simulink model "amp_qpsk"  (Simulink 6.0)
settings: Solver=FixedStepDiscrete  StartTime=0.0  StopTime=10.0  RelTol=1e-3
undefined symbols (not defined in the file or in its folder): read, rfdata
libraries: rfports1 x2, commfilt2 x2, commsink2 x2, rfamplifiers1 x1, commdigbbndpm2 x1, commrandsrc2 x1, simulink x1
settings Model: Creator=ashivapr  LastModifiedBy=fwei  ProdHWDeviceType=Specified
settings DataIOCC: SaveOutput=off  SaveTime=off  SignalLoggingName=logsOut
settings DebuggingCC: CheckExecutionContextPreStartOutputMsg=on  CheckExecutionContextRuntimeOutputMsg=on  SolverPrmCheckMsg=none  InheritedTsInSrcMsg=none
settings HardwareCC: ProdHWDeviceType=Specified
settings ModelReferenceCC: UpdateModelReferenceTargets=IfOutOfDate

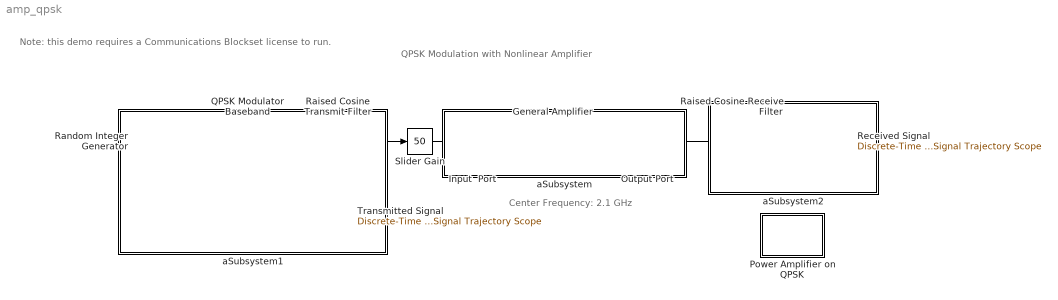
== system amp_qpsk ==
  note: QPSK Modulation with Nonlinear Amplifier
  note: Center Frequency: 2.1 GHz
  note: Note: this demo requires a
      | Communications Blockset
      | license to run.
  General Amplifier : rfamplifiers1/General Amplifier  PhysicalDomain=rfsystemsdomain  SubClassName=general-amplifier  LeftPortType=p1  RightPortType=p1  LConnTagsString=__newl0  RConnTagsString=__newr0  RFDATA=read(rfdata.data, 'default.amp')  InterpMethod=Cubic  IP3Type=OIP3  IIP3=inf  OIP3=inf  NF=0  DisplayData=off  PlotFreq=Derived from Input Port parameters  PlotFreqNoSim=Extracted from RFDATA object  Freq=[1.0e9:1.0e8:2.9e9]  AllPlotType=X-Y plane  NetworkData=S21  PowerData=S11  SmithData=S11  PolarData=S11  ComplexFormat=Magnitude (decibels)  DBFormat=Magnitude (decibels)  PowerFormat=dBm  PhaseFormat=Angle (degrees)  NoneFormat=None
  Input  Port : rfports1/Input Port  Description=source block  MaxLength=128  Fc=2.1e9  Ts=3e-9/8  Zs=50  NoiseFlag=off  seed=67987  GoToTag=AABDAKNBHBUINLASQGFHOGA
  Output Port : rfports1/Output Port  Zl=50  num_Models=3  GoToTag=AABDAKNBHBUINLASQGFHOGA  DisplayData=off  PlotFreq=Derived from Input Port parameters  Freq=1e9:1e8:3e9  AllPlotType=Composite data  NoBudgetPlot=Composite data  NetworkData=S11  SmithData=S11  PolarData=S11  ComplexFormat=Magnitude (decibels)  DBFormat=Magnitude (decibels)  DBMFormat=dBm  NoneFormat=None
  Power Amplifier on QPSK : Subsystem  PropExecContextAcrossSSBoundary=on
      mask Display: disp('Info')
  QPSK Modulator Baseband : commdigbbndpm2/QPSK Modulator Baseband  InType=Integer  Enc=Binary  Ph=pi/4  numSamp=1
  Raised Cosine Receive Filter : commfilt2/Raised Cosine Receive Filter  filtType=Square root  N=8  D=4  R=0.2  sampMode=Frame-based  rateMode=Downsampling  downFactor=8  downOffset=0  checkGain=Normalized  filterGain=1  checkCoeff=off  variableName=rcRxFilt  launchFVT=off
  Raised Cosine Transmit Filter : commfilt2/Raised Cosine Transmit Filter  filtType=Square root  D=4  R=0.2  sampMode=Frame-based  N=8  checkGain=Normalized  filterGain=1  checkCoeff=off  variableName=rcTxFilt  launchFVT=off
  Random Integer Generator : commrandsrc2/Random Integer Generator  mul=4  seed=37  Ts=3e-9  frameBased=on  sampPerFrame=256  orient=off
  Received Signal : commsink2/Discrete-Time Signal Trajectory Scope  Tag=SignalTrajectory  sampPerSymb=1  offsetEye=0  numTraces=40  numNewFrames=10  LineStyles=-  LineColors=b  fading=on  render=on  AxisGrid=on  xMin=-37.4427331807026  xMax=36.8743828925769  yMin=-37.7033821591145  yMax=36.6137339141651  inphaseLabel=In-phase Amplitude  quadratureLabel=Quadrature Amplitude  openScopeAtSimStart=on  FrameNumber=off  FigPos=[393 295 323 323]  figTitle=Signal Trajectory  numLinesMax=8  block_type_=xy
  Slider Gain : simulink/Math Operations/Slider Gain  low=0.1  gain=50  high=100
  Transmitted Signal : commsink2/Discrete-Time Signal Trajectory Scope  Tag=SignalTrajectory  sampPerSymb=1  offsetEye=0  numTraces=40  numNewFrames=10  LineStyles=-  LineColors=b  fading=on  render=on  AxisGrid=on  xMin=-0.777817459305202  xMax=0.781352993211135  yMin=-0.777817459305202  yMax=0.781352993211135  inphaseLabel=In-phase Amplitude  quadratureLabel=Quadrature Amplitude  openScopeAtSimStart=on  FrameNumber=off  FigPos=[41 274 344 344]  figTitle=Signal Trajectory  numLinesMax=8  block_type_=xy
  aSubsystem : Subsystem  PropExecContextAcrossSSBoundary=on
      mask Display: disp('')
  aSubsystem1 : Subsystem  PropExecContextAcrossSSBoundary=on
      mask Display: disp('')
  aSubsystem2 : Subsystem  PropExecContextAcrossSSBoundary=on
      mask Display: disp('')
  wires:
  Raised Cosine Transmit Filter/1 -> Slider Gain/1
  Random Integer Generator/1 -> QPSK Modulator Baseband/1
  Output Port/1 -> Raised Cosine Receive Filter/1
  Raised Cosine Receive Filter/1 -> Received Signal/1
  QPSK Modulator Baseband/1 -> Transmitted Signal/1, Raised Cosine Transmit Filter/1
  Slider Gain/1 -> Input  Port/1
  connections:
  Input  Port/RConn1 -- General Amplifier/LConn1
  General Amplifier/RConn1 -- Output Port/LConn1

== system amp_qpsk/Power Amplifier on QPSK ==
  note: Effects of Power Amplifier on QPSK Modulation
      |
      | This model illustrates the effects of having a non-linear
      | power amplifier in a communication system.
      |
      | Compression is caused when the instantaneous power levels
      | are too high, leading to saturation of the amplifier. Compression
      | causes clipping and distortion of the modulated signal. The
      | Signal Trajectory plots clearly show the presence
      | of compression.
      |
      | Double click the "Slider Gain" block to change the magnitude
      | of the input signal.

== system amp_qpsk/aSubsystem ==

== system amp_qpsk/aSubsystem1 ==

== system amp_qpsk/aSubsystem2 ==
